simulink model "untitled"  (Simulink 7.6)
settings: Solver=ode45  StartTime=0.01  StopTime=1  RelTol=1e-3
settings Model: Creator=Administrator  LastModifiedBy=Administrator

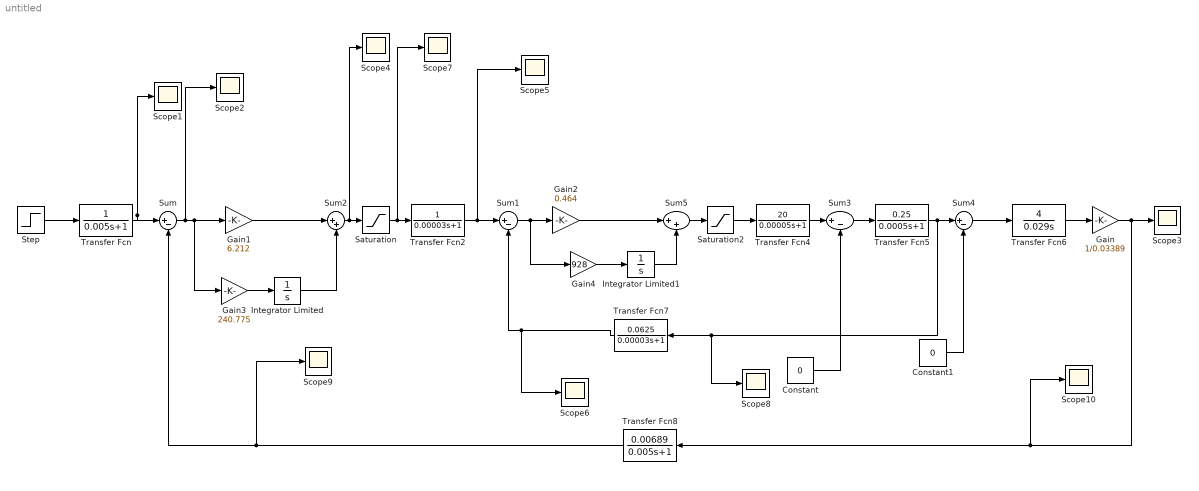
== system untitled ==
  Constant : Constant  Value=0
  Constant1 : Constant  Value=0
  Gain : Gain  Gain=1/0.03389
  Gain1 : Gain  Gain=6.212
  Gain2 : Gain  Gain=0.464
  Gain3 : Gain  Gain=240.775
  Gain4 : Gain  Gain=928
  Integrator Limited : Integrator  LimitOutput=on  UpperSaturationLimit=1  LowerSaturationLimit=0
  Integrator Limited1 : Integrator  LimitOutput=on  UpperSaturationLimit=1  LowerSaturationLimit=0
  Saturation : Saturate  UpperLimit=10  LowerLimit=-10
  Saturation2 : Saturate  UpperLimit=1  LowerLimit=-1
  Scope{1..10} (10 alike) : Scope
      Scope10 settings: SaveName=ScopeData9
      Scope3 settings: TimeRange=0.99  YMin=5250  YMax=8000  SaveName=ScopeData3
      Scope4 settings: SaveName=ScopeData4
      Scope5 settings: SaveName=ScopeData5
      Scope6 settings: SaveName=ScopeData2
      Scope7 settings: SaveName=ScopeData7
      Scope8 settings: SaveName=ScopeData6
      Scope9 settings: SaveName=ScopeData8
  Step : Step  Time=0.1  After=10  SampleTime=0
  Sum{,1,3..4} (4 alike) : Sum  Inputs=|+-
  Sum2 : Sum  Inputs=|++
  Sum5 : Sum  Inputs=|++
  Transfer Fcn : TransferFcn  Denominator=[0.005 1]
  Transfer Fcn2 : TransferFcn  Denominator=[0.00003 1]
  Transfer Fcn4 : TransferFcn  Numerator=[20]  Denominator=[0.00005 1]
  Transfer Fcn5 : TransferFcn  Numerator=[0.25]  Denominator=[0.0005 1]
  Transfer Fcn6 : TransferFcn  Numerator=[4]  Denominator=[0.029 0]
  Transfer Fcn7 : TransferFcn  Numerator=[0.0625]  Denominator=[0.00003 1]
  Transfer Fcn8 : TransferFcn  Numerator=[0.00689]  Denominator=[0.005 1]
  wires:
  Step/1 -> Transfer Fcn/1
  Saturation/1 -> Transfer Fcn2/1, Scope7/1
  Transfer Fcn2/1 -> Sum1/1, Scope5/1
  Transfer Fcn4/1 -> Sum3/1
  Sum3/1 -> Transfer Fcn5/1
  Transfer Fcn5/1 -> Sum4/1, Transfer Fcn7/1, Scope8/1
  Sum4/1 -> Transfer Fcn6/1
  Transfer Fcn6/1 -> Gain/1
  Gain/1 -> Scope3/1, Transfer Fcn8/1, Scope10/1
  Sum/1 -> Gain1/1, Gain3/1, Scope2/1
  Gain1/1 -> Sum2/1
  Sum2/1 -> Saturation/1, Scope4/1
  Transfer Fcn7/1 -> Sum1/2, Scope6/1
  Sum1/1 -> Gain2/1, Gain4/1
  Gain2/1 -> Sum5/1
  Saturation2/1 -> Transfer Fcn4/1
  Sum5/1 -> Saturation2/1
  Constant/1 -> Sum3/2
  Constant1/1 -> Sum4/2
  Transfer Fcn8/1 -> Scope9/1, Sum/2
  Transfer Fcn/1 -> Scope1/1, Sum/1
  Gain3/1 -> Integrator Limited/1
  Integrator Limited/1 -> Sum2/2
  Gain4/1 -> Integrator Limited1/1
  Integrator Limited1/1 -> Sum5/2
